simulink model "OSWEC"  (R2020a)
settings: Solver=ode4  StartTime=0  StopTime=200  FixedStep=0.01  MaxStep=0.01  RelTol=1e-3  EnableMultiTasking=on
values from neighbouring files (symbols this model uses):
  Bv = viscLDamp + ptoDamp + viscQDamp    [ptoSimInputFile.m]    (also in userDefinedFunctions.m)
  controller = struct()    [ptoSimInputFile.m]
  ptosim = ptoSimClass('Non-Compressible Fluid Hydraulic')    [ptoSimInputFile.m]
  R = body(1).hydroData.hydro_coeffs.radiation_damping.all(5,5,w_ind).*simu.rho*2*pi/waves.T    [ptoSimInputFile.m]    (also in userDefinedFunctions.m)
  simu = simulationClass()    [wecSimInputFile.m]
  waves = waveClass('irregular')    [wecSimInputFile.m]
undefined symbols (not defined in the file or in its folder): body, constraint, pto, X, Y, Z
libraries: nesl_utility x22, sm_lib x16, WECSim_Lib x10, PTOSim_Lib x3, vrlib x1, simulink x1
(part 3 of 4)

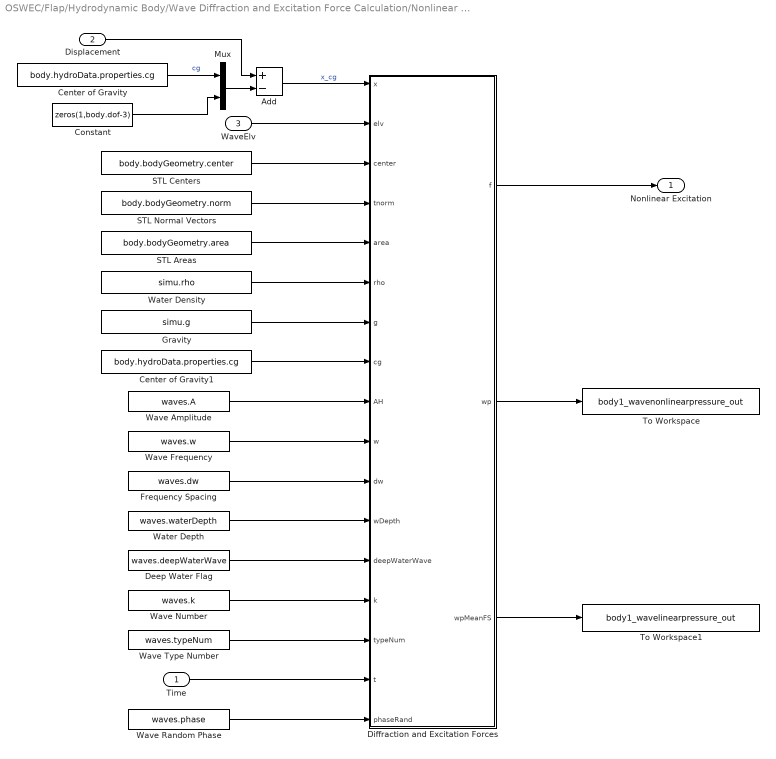
== system OSWEC/Flap/Hydrodynamic Body/Wave Diffraction and Excitation Force Calculation/Nonlinear FK Force Variant Subsystem/With Nonlinear FroudeKrylov Force ==
  Time : Inport
  Displacement : Inport  Port=2
  WaveElv : Inport  Port=3
  Add : Sum  Inputs=+-
  Center of Gravity : Constant  Value=body.hydroData.properties.cg
  Center of Gravity1 : Constant  Value=body.hydroData.properties.cg
  Constant : Constant  Value=zeros(1,body.dof-3)
  Deep Water Flag : Constant  Value=waves.deepWaterWave
  Diffraction and Excitation Forces : MATLAB Function  TreatAsAtomicUnit=on
  Frequency Spacing : Constant  Value=waves.dw
  Gravity : Constant  Value=simu.g
  Mux : Mux  Inputs=2
  STL Areas : Constant  Value=body.bodyGeometry.area
  STL Centers : Constant  Value=body.bodyGeometry.center
  STL Normal Vectors : Constant  Value=body.bodyGeometry.norm
  To Workspace : ToWorkspace  VariableName=body1_wavenonlinearpressure_out  SaveFormat=Structure With Time  SampleTime=-1
      settings: Decimation=round(simu.dtOut/simu.dt,0)
  To Workspace1 : ToWorkspace  VariableName=body1_wavelinearpressure_out  SaveFormat=Structure With Time  SampleTime=-1
      settings: Decimation=round(simu.dtOut/simu.dt,0)
  Water Density : Constant  Value=simu.rho
  Water Depth : Constant  Value=waves.waterDepth
  Wave Amplitude : Constant  Value=waves.A
  Wave Frequency : Constant  Value=waves.w
  Wave Number : Constant  Value=waves.k
  Wave Random Phase : Constant  Value=waves.phase
  Wave Type Number : Constant  Value=waves.typeNum
  Nonlinear Excitation : Outport
  wires:
  STL Areas/1 -> Diffraction and Excitation Forces/5(area)
  Diffraction and Excitation Forces/2(wp) -> To Workspace/1
  Diffraction and Excitation Forces/3(wpMeanFS) -> To Workspace1/1
  Displacement/1 -> Add/1
  Constant/1 -> Mux/2
  Center of Gravity/1 -> Mux/1  "cg"
  Mux/1 -> Add/2
  Add/1 -> Diffraction and Excitation Forces/1(x)  "x_cg"
  Deep Water Flag/1 -> Diffraction and Excitation Forces/13(deepWaterWave)
  Wave Random Phase/1 -> Diffraction and Excitation Forces/17(phaseRand)
  Water Depth/1 -> Diffraction and Excitation Forces/12(wDepth)
  Wave Number/1 -> Diffraction and Excitation Forces/14(k)
  Wave Type Number/1 -> Diffraction and Excitation Forces/15(typeNum)
  Frequency Spacing/1 -> Diffraction and Excitation Forces/11(dw)
  Wave Frequency/1 -> Diffraction and Excitation Forces/10(w)
  Wave Amplitude/1 -> Diffraction and Excitation Forces/9(AH)
  Time/1 -> Diffraction and Excitation Forces/16(t)
  WaveElv/1 -> Diffraction and Excitation Forces/2(elv)
  STL Centers/1 -> Diffraction and Excitation Forces/3(center)
  STL Normal Vectors/1 -> Diffraction and Excitation Forces/4(tnorm)
  Water Density/1 -> Diffraction and Excitation Forces/6(rho)
  Gravity/1 -> Diffraction and Excitation Forces/7(g)
  Diffraction and Excitation Forces/1(f) -> Nonlinear Excitation/1
  Center of Gravity1/1 -> Diffraction and Excitation Forces/8(cg)

== system OSWEC/Flap/Hydrodynamic Body/Wave Radiation Forces Calculation/SS CI and Constant-Damping-CoeVariant Subsystem/Constant Coefficients ==
  note: F = damping * velocity
  velocity : Inport
  Product : Product  Multiplication=Matrix(*)
  Radiation Damping Matrix : Constant  Value=body.hydroForce.fDamping
  Out1 : Outport
  wires:
  velocity/1 -> Product/2
  Product/1 -> Out1/1  "F_Single Frequency"
  Radiation Damping Matrix/1 -> Product/1

== system OSWEC/Flap/Hydrodynamic Body/Wave Radiation Forces Calculation/SS CI and Constant-Damping-CoeVariant Subsystem/Convolution Integral Calculation ==
  note: Calculate the convolution integral using the radiation IRF (body.hydroForce.irkb) and the velocity.
  velocity : Inport
  CTTime : Constant  Value=simu.CTTime
  IRBK : Constant  Value=body.hydroForce.irkb
  MATLAB Function1 : MATLAB Function  TreatAsAtomicUnit=on  SystemSampleTime=simu.CTTime(2)-simu.CTTime(1)
  Rate Transition : RateTransition
  Reshape : Reshape
  Out1 : Outport
  wires:
  velocity/1 -> MATLAB Function1/1(velocity)
  CTTime/1 -> MATLAB Function1/3(CTTime)
  IRBK/1 -> MATLAB Function1/2(IRKB)
  MATLAB Function1/1(F_FM) -> Rate Transition/1
  Rate Transition/1 -> Reshape/1
  Reshape/1 -> Out1/1

== system OSWEC/Flap/Hydrodynamic Body/Wave Radiation Forces Calculation/SS CI and Constant-Damping-CoeVariant Subsystem/State-Space Calculation  ==
  note: Calculate the radiation damping based on the state space formulation. Coefficients are defined in body.hydroForce.ssRadf
  velocity : Inport
  State-Space : StateSpace  A=body.hydroForce.ssRadf.A  B=body.hydroForce.ssRadf.B  C=body.hydroForce.ssRadf.C  D=body.hydroForce.ssRadf.D  InitialCondition=0
  Out1 : Outport
  wires:
  State-Space/1 -> Out1/1
  velocity/1 -> State-Space/1  "x"

== system OSWEC/controller(1)/Rotary to Linear Adjustable Rod1/Angle Calculation for PTO/Subsystem1/Distance btw flap joint & rod joint along x-axis ==
  Add3 : Sum  Inputs=+-
  Add4 : Sum  Inputs=+-
  Constant1 : Constant  Value=ptosim.crank
  Constant2 : Constant  Value=ptosim.rodInit
  Constant3 : Constant  Value=ptosim.offset
  Math Function2 : Math  Operator=square  SignedPower=on  SaturateOnIntegerOverflow=on
  Math Function3 : Math  Operator=square  SignedPower=on  SaturateOnIntegerOverflow=on
  Sqrt1 : Sqrt  SaturateOnIntegerOverflow=on
  d : Outport
  wires:
  Add3/1 -> Sqrt1/1
  Constant2/1 -> Math Function2/1
  Constant1/1 -> Add4/1
  Constant3/1 -> Add4/2
  Add4/1 -> Math Function3/1
  Math Function3/1 -> Add3/2
  Math Function2/1 -> Add3/1
  Sqrt1/1 -> d/1

== system OSWEC/controller(1)/Rotary to Linear Adjustable Rod1/Angle Calculation for PTO/Subsystem2/Distance btw flap joint & rod joint along x-axis ==
  Add3 : Sum  Inputs=+-
  Add4 : Sum  Inputs=+-
  Constant1 : Constant  Value=ptosim.crank
  Constant2 : Constant  Value=ptosim.rodInit
  Constant3 : Constant  Value=ptosim.offset
  Math Function2 : Math  Operator=square  SignedPower=on  SaturateOnIntegerOverflow=on
  Math Function3 : Math  Operator=square  SignedPower=on  SaturateOnIntegerOverflow=on
  Sqrt1 : Sqrt  SaturateOnIntegerOverflow=on
  d : Outport
  wires:
  Add3/1 -> Sqrt1/1
  Constant2/1 -> Math Function2/1
  Constant1/1 -> Add4/1
  Constant3/1 -> Add4/2
  Add4/1 -> Math Function3/1
  Math Function3/1 -> Add3/2
  Math Function2/1 -> Add3/1
  Sqrt1/1 -> d/1

== system OSWEC/controller(1)/Rotary to Linear Adjustable Rod1/Angular to Linear Velocity/Subsystem/Distance btw flap joint & rod joint along x-axis ==
  Add3 : Sum  Inputs=+-
  Add4 : Sum  Inputs=+-
  Constant4 : Constant  Value=ptosim.rodInit
  Constant5 : Constant  Value=ptosim.crank
  Constant6 : Constant  Value=ptosim.offset
  Math Function2 : Math  Operator=square  SignedPower=on  SaturateOnIntegerOverflow=on
  Math Function3 : Math  Operator=square  SignedPower=on  SaturateOnIntegerOverflow=on
  Sqrt1 : Sqrt  SaturateOnIntegerOverflow=on
  d : Outport
  wires:
  Sqrt1/1 -> d/1
  Math Function2/1 -> Add3/1
  Math Function3/1 -> Add3/2
  Add4/1 -> Math Function3/1
  Constant6/1 -> Add4/2
  Constant5/1 -> Add4/1
  Constant4/1 -> Math Function2/1
  Add3/1 -> Sqrt1/1

== system OSWEC/Flap/Hydrodynamic Body/Hydrostatic Restoring Force Calculation/Linear and Nonlinear Restoring Force Variant Subsystem/Linear Hydrostatic Restoring Force /Net Buoyancy Force ==
  note: The total buoyancy force is due to the vertical buoyancy force (gravity - buoyancy) and a rotational buoyancy force if the center of gravity is not aligned with the center of buoyancy.
      |
      | F_NetBuoyancy = F_gravity - F_buoyancy + F_rotational_buoyancy
      |
      | F_rotational_buoyancy = (cb-cg) x F_buoyancy
      | F_buoyancy = rho*g*V_0
      | F_gravity = m*g
  Body Mass : Inport
  Add1 : Sum  Inputs=+-
  Add2 : Sum
  Add3 : Sum  Inputs=+-
  Assignment (Add Net Bouyancy Force to Z-Direction) : Assignment  IndexOptions=Index vector (dialog)  Indices=3  OutputSizes=1
  Assignment (Add Net Bouyancy Force to Z-Direction)1 : Assignment  IndexOptions=Index vector (dialog)  Indices=3  OutputSizes=1
  Assignment (Add Net Bouyancy Force to Z-Direction)2 : Assignment  IndexOptions=Index vector (dialog)  Indices=4:6  OutputSizes=1
  Center of Buoyancy : Constant  Value=body.cb
  Center of Gravity : Constant  Value=body.cg
  Constant1 : Constant  Value=zeros(1,body.dof)
  Constant2 : Constant  Value=[0 0 0]
  Cross Product : vrlib/Utilities/Cross Product
  Gravity : Constant  Value=simu.g
  Product : Product
  Product1 : Product  Inputs=3
  Volume : Constant  Value=body.dispVol
  Water Density : Constant  Value=simu.rho
  F_NetBuoyancy : Outport
  wires:
  Add1/1 -> Assignment (Add Net Bouyancy Force to Z-Direction)/2
  Body Mass/1 -> Product/2  "m"
  Cross Product/1 -> Assignment (Add Net Bouyancy Force to Z-Direction)2/2
  Add2/1 -> F_NetBuoyancy/1  "Net buoyancy force"
  Add3/1 -> Cross Product/2
  Constant2/1 -> Assignment (Add Net Bouyancy Force to Z-Direction)1/1
  Center of Gravity/1 -> Add3/2  "cg"
  Constant1/1 -> Assignment (Add Net Bouyancy Force to Z-Direction)/1, Assignment (Add Net Bouyancy Force to Z-Direction)2/1
  Center of Buoyancy/1 -> Add3/1  "x"
  Assignment (Add Net Bouyancy Force to Z-Direction)1/1 -> Cross Product/1
  Volume/1 -> Product1/3  "Vol"
  Assignment (Add Net Bouyancy Force to Z-Direction)/1 -> Add2/1  "Vertical Buoyancy Force"
  Water Density/1 -> Product1/1  "rho"
  Gravity/1 -> Product/1, Product1/2  "g"
  Product1/1 -> Assignment (Add Net Bouyancy Force to Z-Direction)1/2, Add1/2  "F_Buoyancy"
  Product/1 -> Add1/1  "F_Gravity"
  Assignment (Add Net Bouyancy Force to Z-Direction)2/1 -> Add2/2  "Rotational buoyancy force"

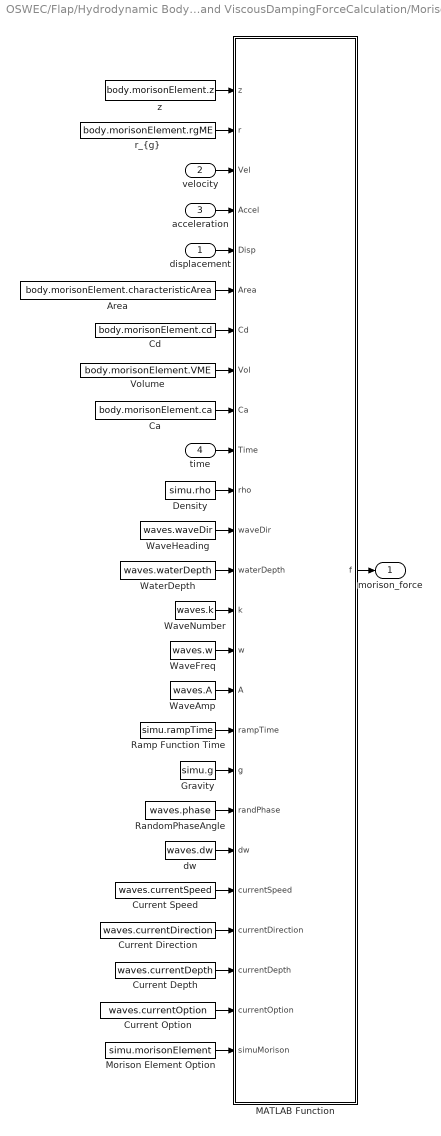
== system OSWEC/Flap/Hydrodynamic Body/Morison Element and ViscousDampingForceCalculation/Morison Element Variant Subsystem/Morison Element On/Irregular Wave Morison Force ==
  displacement : Inport
  velocity : Inport  Port=2
  acceleration : Inport  Port=3
  time : Inport  Port=4
  Area : Constant  Value=body.morisonElement.characteristicArea  VectorParams1D=off
  Ca : Constant  Value=body.morisonElement.ca  VectorParams1D=off
  Cd : Constant  Value=body.morisonElement.cd  VectorParams1D=off
  Current Depth : Constant  Value=waves.currentDepth
  Current Direction : Constant  Value=waves.currentDirection
  Current Option : Constant  Value=waves.currentOption
  Current Speed : Constant  Value=waves.currentSpeed
  Density : Constant  Value=simu.rho
  Gravity : Constant  Value=simu.g
  MATLAB Function : MATLAB Function  TreatAsAtomicUnit=on
  Morison Element Option : Constant  Value=simu.morisonElement
  Ramp Function Time : Constant  Value=simu.rampTime
  RandomPhaseAngle : Constant  Value=waves.phase  VectorParams1D=off
  Volume : Constant  Value=body.morisonElement.VME  VectorParams1D=off
  WaterDepth : Constant  Value=waves.waterDepth
  WaveAmp : Constant  Value=waves.A
  WaveFreq : Constant  Value=waves.w
  WaveHeading : Constant  Value=waves.waveDir
  WaveNumber : Constant  Value=waves.k
  dw : Constant  Value=waves.dw  VectorParams1D=off
  "r_{g}" : Constant  Value=body.morisonElement.rgME  VectorParams1D=off
  z : Constant  Value=body.morisonElement.z  VectorParams1D=off
  morison_force : Outport
  wires:
  Morison Element Option/1 -> MATLAB Function/25(simuMorison)
  Current Option/1 -> MATLAB Function/24(currentOption)
  Current Depth/1 -> MATLAB Function/23(currentDepth)
  Current Direction/1 -> MATLAB Function/22(currentDirection)
  Current Speed/1 -> MATLAB Function/21(currentSpeed)
  dw/1 -> MATLAB Function/20(dw)
  RandomPhaseAngle/1 -> MATLAB Function/19(randPhase)
  Gravity/1 -> MATLAB Function/18(g)
  Ramp Function Time/1 -> MATLAB Function/17(rampTime)
  WaveAmp/1 -> MATLAB Function/16(A)
  WaveFreq/1 -> MATLAB Function/15(w)
  WaveNumber/1 -> MATLAB Function/14(k)
  WaterDepth/1 -> MATLAB Function/13(waterDepth)
  WaveHeading/1 -> MATLAB Function/12(waveDir)
  Density/1 -> MATLAB Function/11(rho)
  time/1 -> MATLAB Function/10(Time)
  Ca/1 -> MATLAB Function/9(Ca)
  Volume/1 -> MATLAB Function/8(Vol)
  Cd/1 -> MATLAB Function/7(Cd)
  Area/1 -> MATLAB Function/6(Area)
  displacement/1 -> MATLAB Function/5(Disp)
  acceleration/1 -> MATLAB Function/4(Accel)
  velocity/1 -> MATLAB Function/3(Vel)
  "r_{g}"/1 -> MATLAB Function/2(r)
  z/1 -> MATLAB Function/1(z)
  MATLAB Function/1(f) -> morison_force/1

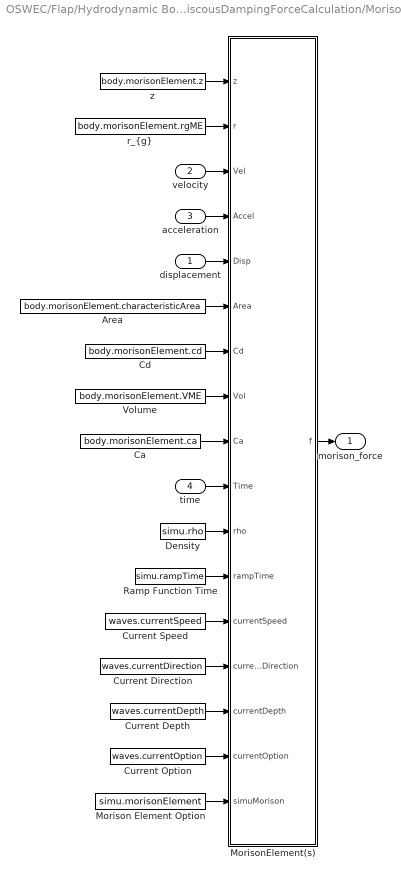
== system OSWEC/Flap/Hydrodynamic Body/Morison Element and ViscousDampingForceCalculation/Morison Element Variant Subsystem/Morison Element On/No Wave Morison Force ==
  displacement : Inport
  velocity : Inport  Port=2
  acceleration : Inport  Port=3
  time : Inport  Port=4
  Area : Constant  Value=body.morisonElement.characteristicArea  VectorParams1D=off
  Ca : Constant  Value=body.morisonElement.ca  VectorParams1D=off
  Cd : Constant  Value=body.morisonElement.cd  VectorParams1D=off
  Current Depth : Constant  Value=waves.currentDepth
  Current Direction : Constant  Value=waves.currentDirection
  Current Option : Constant  Value=waves.currentOption
  Current Speed : Constant  Value=waves.currentSpeed
  Density : Constant  Value=simu.rho
  Morison Element Option : Constant  Value=simu.morisonElement
  MorisonElement(s) : MATLAB Function  TreatAsAtomicUnit=on
  Ramp Function Time : Constant  Value=simu.rampTime
  Volume : Constant  Value=body.morisonElement.VME  VectorParams1D=off
  "r_{g}" : Constant  Value=body.morisonElement.rgME  VectorParams1D=off
  z : Constant  Value=body.morisonElement.z  VectorParams1D=off
  morison_force : Outport
  wires:
  Morison Element Option/1 -> MorisonElement(s)/17(simuMorison)
  Current Option/1 -> MorisonElement(s)/16(currentOption)
  Current Depth/1 -> MorisonElement(s)/15(currentDepth)
  Current Direction/1 -> MorisonElement(s)/14(currentDirection)
  Current Speed/1 -> MorisonElement(s)/13(currentSpeed)
  Ramp Function Time/1 -> MorisonElement(s)/12(rampTime)
  Density/1 -> MorisonElement(s)/11(rho)
  time/1 -> MorisonElement(s)/10(Time)
  Ca/1 -> MorisonElement(s)/9(Ca)
  Volume/1 -> MorisonElement(s)/8(Vol)
  Cd/1 -> MorisonElement(s)/7(Cd)
  Area/1 -> MorisonElement(s)/6(Area)
  displacement/1 -> MorisonElement(s)/5(Disp)
  acceleration/1 -> MorisonElement(s)/4(Accel)
  velocity/1 -> MorisonElement(s)/3(Vel)
  "r_{g}"/1 -> MorisonElement(s)/2(r)
  z/1 -> MorisonElement(s)/1(z)
  MorisonElement(s)/1(f) -> morison_force/1

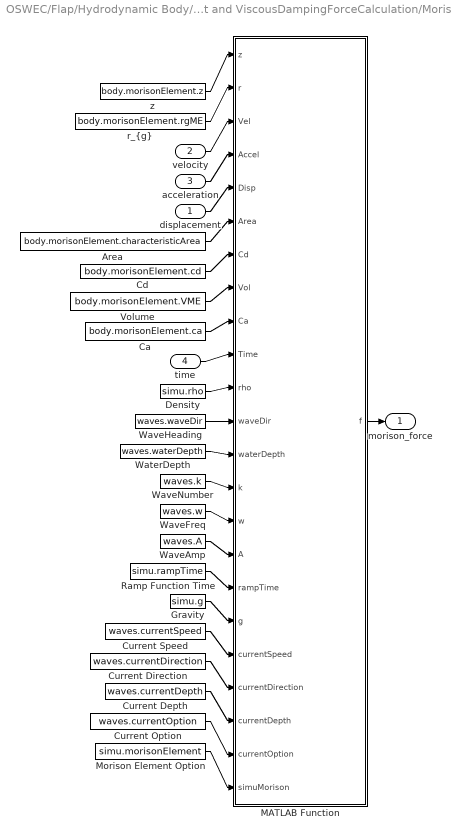
== system OSWEC/Flap/Hydrodynamic Body/Morison Element and ViscousDampingForceCalculation/Morison Element Variant Subsystem/Morison Element On/Regular Wave Morison Force ==
  displacement : Inport
  velocity : Inport  Port=2
  acceleration : Inport  Port=3
  time : Inport  Port=4
  Area : Constant  Value=body.morisonElement.characteristicArea  VectorParams1D=off
  Ca : Constant  Value=body.morisonElement.ca  VectorParams1D=off
  Cd : Constant  Value=body.morisonElement.cd  VectorParams1D=off
  Current Depth : Constant  Value=waves.currentDepth
  Current Direction : Constant  Value=waves.currentDirection
  Current Option : Constant  Value=waves.currentOption
  Current Speed : Constant  Value=waves.currentSpeed
  Density : Constant  Value=simu.rho
  Gravity : Constant  Value=simu.g
  MATLAB Function : MATLAB Function  TreatAsAtomicUnit=on
  Morison Element Option : Constant  Value=simu.morisonElement
  Ramp Function Time : Constant  Value=simu.rampTime
  Volume : Constant  Value=body.morisonElement.VME  VectorParams1D=off
  WaterDepth : Constant  Value=waves.waterDepth
  WaveAmp : Constant  Value=waves.A
  WaveFreq : Constant  Value=waves.w
  WaveHeading : Constant  Value=waves.waveDir
  WaveNumber : Constant  Value=waves.k
  "r_{g}" : Constant  Value=body.morisonElement.rgME  VectorParams1D=off
  z : Constant  Value=body.morisonElement.z  VectorParams1D=off
  morison_force : Outport
  wires:
  Current Speed/1 -> MATLAB Function/19(currentSpeed)
  WaveAmp/1 -> MATLAB Function/16(A)
  Gravity/1 -> MATLAB Function/18(g)
  WaveNumber/1 -> MATLAB Function/14(k)
  Ca/1 -> MATLAB Function/9(Ca)
  Current Direction/1 -> MATLAB Function/20(currentDirection)
  Area/1 -> MATLAB Function/6(Area)
  WaterDepth/1 -> MATLAB Function/13(waterDepth)
  acceleration/1 -> MATLAB Function/4(Accel)
  Density/1 -> MATLAB Function/11(rho)
  WaveHeading/1 -> MATLAB Function/12(waveDir)
  WaveFreq/1 -> MATLAB Function/15(w)
  Cd/1 -> MATLAB Function/7(Cd)
  displacement/1 -> MATLAB Function/5(Disp)
  Current Option/1 -> MATLAB Function/22(currentOption)
  Current Depth/1 -> MATLAB Function/21(currentDepth)
  time/1 -> MATLAB Function/10(Time)
  "r_{g}"/1 -> MATLAB Function/2(r)
  Ramp Function Time/1 -> MATLAB Function/17(rampTime)
  velocity/1 -> MATLAB Function/3(Vel)
  Volume/1 -> MATLAB Function/8(Vol)
  Morison Element Option/1 -> MATLAB Function/23(simuMorison)
  z/1 -> MATLAB Function/1(z)
  MATLAB Function/1(f) -> morison_force/1

== matlab function OSWEC/Flap/Hydrodynamic Body/Morison Element and ViscousDampingForceCalculation/Morison Element Variant Subsystem/Morison Element On/Irregular Wave Morison Force/MATLAB Function ==
  data: z input; f output; r input; Vel input; Accel input; Disp input; Area input; Cd input; Vol input; Ca input; Time input; rho input; waveDir input; waterDepth input; k input; w input; A input; rampTime input; g input; randPhase input; dw input; currentSpeed input; currentDirection input; currentDepth input; currentOption input; simuMorison input
function f = fcn(z,r,Vel,Accel,Disp,Area,Cd,Vol,Ca,Time,rho,waveDir,waterDepth,k,w,A,rampTime,g,randPhase,dw,currentSpeed,currentDirection,currentDepth,currentOption,simuMorison)
% This function calculates the Morison element force for the irregular wave
% case.
[rr,~]  = size(r); [ff]    = length(w);
FMt     = zeros(rr,6);
uVt     = zeros(ff,1); vVt = uVt; wVt = vVt; uAt = wVt; vAt = uAt; wAt = vAt;
for ii = 1:rr
    % Calculate Rotation Matrix
    RotMax = [cos(Disp(5))*cos(Disp(6)) , cos(Disp(4))*sin(Disp(6)) + sin(Disp(4))*sin(Disp(5))*cos(Disp(6)) , sin(Disp(4))*sin(Disp(6)) - cos(Disp(4))*sin(Disp(5))*sin(Disp(6));...
              -cos(Disp(5))*sin(Disp(6)), cos(Disp(4))*cos(Disp(6)) -  sin(Disp(4))*sin(Disp(5))*sin(Disp(6)), sin(Disp(4))*cos(Disp(6)) + cos(Disp(4))*sin(Disp(5))*sin(Disp(6));...
              sin(Disp(5))              , -sin(Disp(4))*cos(Disp(5))                                         , cos(Disp(4))*cos(Disp(5))                                        ];
    % Rotate Cartesian
    rRot    = mtimes(RotMax,r(ii,:).')';
    Dispt   = [Disp(1),Disp(2),Disp(3)];
    ShiftCg = Dispt + rRot;
    zRot    = mtimes(RotMax,z(ii,:)')';
    % Update translational and rotational velocity
    % w refers to \omega = rotational velocity
    Velt    = [Vel(4),Vel(5),Vel(6)];
    wxr     = cross(Velt,r(ii,:));
    %
    switch currentOption
        case 0
            currentSpeedDepth = currentSpeed;
        case 1
            if ShiftCg(3) > -currentDepth
                currentSpeedDepth = currentSpeed*(1 + ShiftCg(3)/currentDepth)^(1/7);
            else
                currentSpeedDepth = 0;
            end
        case 2
            if ShiftCg(3) > -currentDepth
                currentSpeedDepth = currentSpeed*(1 + ShiftCg(3)/currentDepth);
            else
                currentSpeedDepth = 0;
            end
        otherwise
            currentSpeedDepth = 0;
    end
    % Ramp Time
    if Time <= rampTime
        curramp        = currentSpeedDepth*(1 + cos(pi + pi/rampTime*Time))/2;
    else
        curramp        = currentSpeedDepth;
    end
    %Vel should be a column vector
    Vel2    = [Vel(1),Vel(2),Vel(3)] + wxr + [curramp*cosd(currentDirection),curramp*sind(currentDirection),0];
    % Update translational and rotational acceleration
    % dotw refers to \dot{\omega} = rotational acceleration
    Accelt  = [Accel(4),Accel(5),Accel(6)];
    dotwxr  = cross(Accelt,r(ii,:));
    wxwxr   = cross(Velt,wxr);
    % Update Translational Acceleration
    Accel2  = [Accel(1),Accel(2),Accel(3)] + dotwxr + wxwxr;
    %% Calculate Orbital Velocity
    for jj = 1:ff
        waveDirRad      = waveDir*pi/180;
        phaseArg        = w(jj,1)*Time - k(jj,1)*(ShiftCg(1)*cos(waveDirRad) + ShiftCg(2)*sin(waveDirRad)) + randPhase(jj,1);
        % Vertical Variation
        kh              = k(jj,1)*waterDepth;
        kz              = k(jj,1)*ShiftCg(3);
        if kh > pi 
            % Deep Water Wave Assumption
            coeffHorz  = exp(kz);
            coeffVert  = coeffHorz;
        else
            % Shallow & Intermediate depth
            coeffHorz  = cosh(kz + kh)/cosh(kh);
            coeffVert  = sinh(kz + kh)/cosh(kh);
        end
        % Ramp Time
        if Time <= rampTime
            ramp        = (sqrt(A(jj,1)*dw(jj,1))/2)*(1 + cos(pi + pi/rampTime*Time));
        else
            ramp        = sqrt(A(jj,1)*dw(jj,1));
        end
        % Orbital Velocity for each individual wave component
        uVt(jj,1)       =  ramp*coeffHorz*cos(phaseArg)*g*k(jj,1)*(1/w(jj,1))*cos(waveDirRad);
        vVt(jj,1)       =  ramp*coeffHorz*cos(phaseArg)*g*k(jj,1)*(1/w(jj,1))*sin(waveDirRad);
        wVt(jj,1)       = -ramp*coeffVert*sin(phaseArg)*g*k(jj,1)*(1/w(jj,1));
        % Orbital Acceleration for each individual wave component
        uAt(jj,1)       = -ramp*coeffHorz*sin(phaseArg)*g*k(jj,1)*cos(waveDirRad);
        vAt(jj,1)       = -ramp*coeffHorz*sin(phaseArg)*g*k(jj,1)*sin(waveDirRad);
        wAt(jj,1)       = -ramp*coeffVert*cos(phaseArg)*g*k(jj,1);
    end
    % Sum the wave components to obtain the x, y, z orbital velocities
    uV = sum(uVt); uA   = sum(uAt); vV = sum(vVt); vA = sum(vAt); wV = sum(wVt); wA = sum(wAt);
    fluidV              = [uV, vV, wV];
    fluidA              = [uA, vA, wA];
    if simuMorison == 2
        %% Decompose Fluid Velocity
        % Tangential Velocity
        vT              = ((dot(zRot,fluidV))/(norm(zRot)^2))*zRot;        
        % Normal Velocity
        vN              = fluidV-vT;
        %% Decompose Fluid Acceleration
        AT              = ((dot(zRot,fluidA))/(norm(zRot)^2))*zRot;        
        % Normal Acceleration
        AN              = fluidA-AT;
        %% Decompose Body Velocity
        % Tangential Velocity
        Vel2T           = ((dot(zRot,Vel2))/(norm(zRot)^2))*zRot;       
        % Normal Velocity
        Vel2N           = Vel2-Vel2T;
        %% Decompose Body Acceleration
        Accel2T         = ((dot(zRot,Accel2))/(norm(zRot)^2))*zRot;   
        % Normal Acceleration
        Accel2N         = Accel2-Accel2T;
        %% Morison Equation
        % Forces from velocity drag
        FdN             = (1/2)*rho*Cd(ii,1)*Area(ii,1)*(vN-Vel2N)*norm(vN-Vel2N);                               
        FdT             = (1/2)*rho*Cd(ii,2)*Area(ii,2)*(vT-Vel2T)*norm(vT-Vel2T);                                          
        Fd              = FdT + FdN;
        % Forces from body acceleration inertia on the Morison Element
        FiN             = rho*Vol(ii,:)*Ca(ii,1)*(AN - Accel2N);            % AdiffN;
        FiT             = rho*Vol(ii,:)*Ca(ii,2)*(AT - Accel2T);            % AdiffT;
        Fbi             = FiN + FiT;
        % Forces from fluid acceleration inertia on the Morison Element
        Ffi             = rho*Vol(ii,:)*(fluidA);
        % Summation of inertial forces on the Morison Element
        Fi              = Ffi + Fbi;
        % Total Force from the Morison Element
        F               = Fi + Fd;
    else
        %% Added inertia and drag forces
        areaRot         = abs(mtimes(Area(ii,:),RotMax));
        CdRot           = mtimes(abs(Cd(ii,:)),RotMax);
        CaRot           = abs(mtimes(Ca(ii,:),RotMax));
        % Forces from velocity drag
        uVdiff          = uV - Vel2(1); FxuV = (1/2)*abs(uVdiff)*uVdiff*rho*CdRot(1)*areaRot(1);
        vVdiff          = vV - Vel2(2); FxvV = (1/2)*abs(vVdiff)*vVdiff*rho*CdRot(2)*areaRot(2);
        wVdiff          = wV - Vel2(3); FxwV = (1/2)*abs(wVdiff)*wVdiff*rho*CdRot(3)*areaRot(3);
        % Forces from body acceleration inertia
        uAdiff          = uA - Accel2(1); FxuA = uAdiff*rho*Vol(ii,:)*CaRot(1);
        vAdiff          = vA - Accel2(2); FxvA = vAdiff*rho*Vol(ii,:)*CaRot(2);
        wAdiff          = wA - Accel2(3); FxwA = wAdiff*rho*Vol(ii,:)*CaRot(3);
        % Forces from fluid acceleration inertia
        FxuAf           = uA*Vol(ii,:)*rho;
        FxvAf           = vA*Vol(ii,:)*rho;
        FxwAf           = wA*Vol(ii,:)*rho;
        % Total Force from the Morison Element
        F               = [FxuV + FxuA + FxuAf,...
                           FxvV + FxvA + FxvAf,...
                           FxwV + FxwA + FxwAf];
    end
    % Determine if the Morison Element point of application goes above the
    % mean water line and does not consider the local surface elevation.
    if ShiftCg(3) > 0
        F           = [0, 0, 0];
        M           = [0, 0, 0];
        FMt(ii,:)   = [F,M];
    else
        % Calculate the moment about the center of gravity for each Morison Element
        M           = cross(rRot,F);
        FMt(ii,:)   = [F,M];
    end
end
f      = 0.* Vel;
f(1:6) = [sum(FMt(:,1));sum(FMt(:,2));sum(FMt(:,3));sum(FMt(:,4));sum(FMt(:,5));sum(FMt(:,6))];

== matlab function OSWEC/Flap/Hydrodynamic Body/Nonlinear Wave Elevation/Linear or Instantaneous Free Surface/Instantaneous Water Free Surface  /Instantaneous FS ==
  data: x input; center input; f output; cg input; AH input; w input; dw input; k input; typeNum input; t input; rampT input; phaseRand input; waveDir input
function f  = waveElevation(x,center,cg,AH,w,dw,k,typeNum,t,rampT,phaseRand,waveDir)
% Function to calculate the wave elevation at the ceontroids of triangulated surface
% NOTE: This function assumes that the STL file is imported with its CG at 0,0,0
f = calc_elev(x,center,cg,AH,w,dw,k,typeNum,t,rampT,phaseRand, waveDir);
end

function f = calc_elev(x,center,cg,AH,w,dw,k,typeNum,t,rampT,phaseRand,waveDir)
% Function to rotate and translate body and call wave elevation function at new locations

% Compute new tri center coords after cog rotation and translation
center = rotateXYZ(center,[1 0 0],x(4));
center = rotateXYZ(center,[0 1 0],x(5));
center = rotateXYZ(center,[0 0 1],x(6));
center = offsetXYZ(center,x);
center = offsetXYZ(center,cg);
% Calculate the free surface
f=waveElev(center,AH,w,dw,t,k,rampT,phaseRand,typeNum,waveDir);
end

function f=waveElev(center,AH,w,dw,t,k,rampT,phaseRand,typeNum,waveDir)
% Function to calculate the wave elevation at an array of points
f = zeros(length(center(:,3)),1);
cx = center(:,1);
cy = center(:,2);
X = cx*cos(waveDir*pi/180) + cy*sin(waveDir*pi/180);
if typeNum <10
elseif typeNum <20
    f = AH(1).*cos(k(1).*X-w(1)*t);
elseif typeNum <30
    tmp=sqrt(AH.*dw);
    tmp1 = ones(1,length(center(:,1)));
    tmp2 = (w.*t+phaseRand)*tmp1;
    tmp3 = cos(k*X'- tmp2);
    f(:,1) = tmp3'*tmp;
end
if t<=rampT
    rampF = (1+cos(pi+pi*t/rampT))/2;
    f = f.*rampF;
end
end

== matlab function OSWEC/Flap/Hydrodynamic Body/Structure/Motion Sensor/quaternion2EulXYZ ==
  data: Q input; E output
function E = fcn(Q)
% Call quaternion matlab function. 
% Saved as separate text file for Github tracking purposes.
% Can't use MATLAB interpreted function because they don't allow for code 
% generation (used in rapid accelerator mode)
E = quaternion2EulXYZ(Q);
end

== matlab function OSWEC/Flap/Hydrodynamic Body/Wave Diffraction and Excitation Force Calculation/Linear Wave Excitation Force Variant Subsystem/Irregular Wave Excitation Force/MATLAB Function ==
  data: A input; Fext output; w input; fExtRE input; fExtIM input; phaseRand input; dw input; time input; WaveDir input; WaveSpread input; fExtMD input
function Fext = fcn(A,w,fExtRE,fExtIM,phaseRand,dw,time,WaveDir,WaveSpread,fExtMD)
%#codegen

% pversistent A1 B1 B11 C1 D1 D11 E1 E11

A1=bsxfun(@plus,w*time,pi/2);
%Fext = zeros(1,6);
Fext = zeros(1,size(fExtRE,3));
for ii=1:length(WaveDir)
    B1= sin(bsxfun(@plus,A1,phaseRand(:,ii)));
    B11 = sin(bsxfun(@plus,w*time,phaseRand(:,ii)));
    C0 = bsxfun(@times,A*WaveSpread(ii),dw);
    C1 = sqrt(bsxfun(@times,A*WaveSpread(ii),dw));
    D0 =bsxfun(@times,squeeze(fExtMD(ii,:,:)),C0);
    D1 =bsxfun(@times,squeeze(fExtRE(ii,:,:)),C1);
    D11 = bsxfun(@times,squeeze(fExtIM(ii,:,:)),C1);
    E1 = D0+ bsxfun(@times,B1,D1);
    E11 = bsxfun(@times,B11,D11);
    Fext = Fext + sum(bsxfun(@minus,E1,E11));
end

== matlab function OSWEC/Flap/Hydrodynamic Body/Wave Diffraction and Excitation Force Calculation/Nonlinear FK Force Variant Subsystem/With Nonlinear FroudeKrylov Force/Diffraction and Excitation Forces ==
  data: x input; elv input; center input; f output; tnorm input; area input; rho input; g input; cg input; AH input; w input; dw input; wDepth input; deepWaterWave input; k input; typeNum input; t input; phaseRand input; wp output; wpMeanFS output
function [f, wp, wpMeanFS]  = nonFKForce(x,elv,center,tnorm,area,rho,g,cg,AH,w,dw,wDepth,deepWaterWave,k,typeNum,t,phaseRand)
% Function to calculate the wave excitation force and moment on a
% triangulated surface. The nonlinear excitation forces are calculated by
% intergrating the pressure over the triangulated surface and subtracting
% the linear excitation force (this is added back in later):
%    F_exc_nonlinear = F_exc_total - F_exc_linear
% NOTE: This function assumes that the STL file is imported with its CG at 0,0,0

% Logic to calculate nonFKForce at reduced sample time
[f, wp, wpMeanFS] = calc_force(x,elv,center,tnorm,area,rho,g,cg,AH,w,dw,wDepth,deepWaterWave,k,typeNum,t,phaseRand);
end

function [f, wp, wpMeanFS]  = calc_force(x,elv,center,tnorm,area,rho,g,cg,AH,w,dw,wDepth,deepWaterWave,k,typeNum,t,phaseRand)
% Function to apply translation and rotation, and calculate forces.

% Compute new tri coords after cog rotation and translation
centerMeanFS = offsetXYZ(center,cg);
avMeanFS     = tnorm .* [area area area];

% Compute new tri coords after cog rotation and translation
center = rotateXYZ(center,[1 0 0],x(4));
center = rotateXYZ(center,[0 1 0],x(5));
center = rotateXYZ(center,[0 0 1],x(6));
center = offsetXYZ(center,x);
center = offsetXYZ(center,cg);
% Compute new normal vectors coords after cog rotation and translation
tnorm = rotateXYZ(tnorm,[1 0 0],x(4));
tnorm = rotateXYZ(tnorm,[0 1 0],x(5));
tnorm = rotateXYZ(tnorm,[0 0 1],x(6));

% Copute area vectors
av = tnorm .* [area area area];

% Calculate the free surface
wpMeanFS=pDis(centerMeanFS,       0,AH,w,dw,wDepth,deepWaterWave,t,k,phaseRand,typeNum,rho,g);
wp      =pDis(center      ,     elv,AH,w,dw,wDepth,deepWaterWave,t,k,phaseRand,typeNum,rho,g);

% Calculate forces
f_linear   =FK(centerMeanFS,       cg,avMeanFS,wpMeanFS);
f_nonLinear=FK(center      ,x(1:3)+cg,av      ,wp      );
f = f_nonLinear-f_linear;
end

function f=pDis(center,elv,AH,w,dw,wDepth,deepWaterWave,t,k,phaseRand,typeNum,rho,g)
% Function to calculate pressure distribution
f = zeros(length(center(:,3)),1);
z=zeros(length(center(:,1)),1);
if typeNum <10
elseif typeNum <20
    f = rho.*g.*AH(1).*cos(k(1).*center(:,1)-w(1)*t);
    if deepWaterWave == 0
        z=(center(:,3)-elv).*wDepth./(wDepth+elv);
        f = f.*(cosh(k(1).*(z+wDepth))./cosh(k(1)*wDepth));
    else
        z=(center(:,3)-elv);
        f = f.*exp(k(1).*z);
    end
elseif typeNum <30
    for i=1:length(AH)
        if deepWaterWave == 0 && wDepth <= 0.5*pi/k(i)
            z=(center(:,3)-elv).*wDepth./(wDepth+elv);
            f_tmp = rho.*g.*sqrt(AH(i)*dw(i)).*cos(k(i).*center(:,1)-w(i)*t-phaseRand(i));
            f = f + f_tmp.*(cosh(k(i).*(z+wDepth))./cosh(k(i).*wDepth));
        else
            z=(center(:,3)-elv);
            f_tmp = rho.*g.*sqrt(AH(i)*dw(i)).*cos(k(i).*center(:,1)-w(i)*t-phaseRand(i));
            f = f + f_tmp.*exp(k(i).*z);
        end
    end
end
f(z>0)=0;
end

function f = FK(center,instcg,av,wp)
% Function to calculate the force and moment about the cog due to Froude-Krylov pressure
f = zeros(6,1);

% Calculate the hydrostatic pressure at each triangle center
pressureVect = [wp wp wp].*-av;

% Compute force about cog
f(1:3) = sum(pressureVect);

% Compute moment about cog
tmp1 = ones(length(center(:,1)),1);
tmp2 = tmp1*instcg';
center2cgVec = center-tmp2;

f(4:6)= sum(cross(center2cgVec,pressureVect));
end

== matlab function OSWEC/Flap/Hydrodynamic Body/Wave Radiation Forces Calculation/SS CI and Constant-Damping-CoeVariant Subsystem/Convolution Integral Calculation/MATLAB Function1 ==
  data: velocity input; F_FM output; IRKB input; CTTime input
function F_FM = ConvolutionIntegral_interp(velocity, IRKB, CTTime)
%#codegen
% Function to calculate convolution integral. velocity is the only dynamic input.
% IRKB, nDOF and CTTime do not change with time.
%
% Dimensions:
% nDOF = the body's number of degrees of freedom = body.dof
% LDOF = radiating dofs from all bodies (6*Nbodies)
% nt = length of CTTime (simu.CITime / simu.dtCTTime)
%
% Paramters:
%     velocity : float [LDOF]
%         The current velocities of all bodies 
%         e.g. 6 for 1 body, 12 for 2 bodies and B2B on
% 
%     IRKB : float [nt nDOF LDOF]
%         The body's interpolated IRF, as calculated in irfInfAddedMassAndDamping
% 
%     CTTime : float [nt]
%         All CI times
%
% Returns:
%     F_FM : float [nDOF,1]

% define persistent variables to track velocity_history over time. Others are
% persistent so that the static values only need be calculated once.
interp_factor = 1;
persistent velocity_history IRKB_interp CTTime_interp;

% If this is the first time step (i.e. velocity_history is empty), 
% define the persistent variables.
if isempty(velocity_history) 
    CTTime_interp  = CTTime(1:interp_factor:end);         % [nt] interpolate CTTime if interpolation timestep ~= 1
    velocity_history = zeros(length(CTTime_interp),length(velocity)); % [nt LDOF]
    irkb_tmp    = IRKB(1:interp_factor:end, :, :);     % [nt nDOF LDOF] interpolate IRKB if interpolation timestep ~= 1
    IRKB_interp = permute(irkb_tmp,[1 3 2]); % permute to [nt LDOF nDOF]
end 

% shift velocity_history to set the first column as the current velocity
velocity_history = circshift(velocity_history, 1, 1); % shift velocity_history by 1 in the time dimension for the new time step
velocity_history(1,:) = velocity(:)';                 % [nt LDOF], fill first row with current velocity

% Multiply velocity_history and IRKB
time_series = bsxfun(@times, IRKB_interp, velocity_history); % [nt LDOF nDOF], multiply velocity_history and K_r for CI integral

% sum the effects of all radiating dofs (LDOF) for each time and motion dof (nDOF)
tmp_s = squeeze(sum(time_series,2)); % [nt nDOF]
F_FM = squeeze(trapz(CTTime_interp,tmp_s,1)); % integrate to get the wave radiation force, [nDOF, 1]

end

== matlab function OSWEC/Flap/Hydrodynamic Body/nonLinYaw force transforms/nonLinYaw force transforms ==
  data: yawNonLin input; F_Excitation output; dispGlobal input; F_RadiationDampingLocal input; F_AddedMassLocal input; F_ExcitationLocal input; F_RadiationDamping output; F_RestoringLocal input; F_AddedMass output; F_Restoring output
function [F_Excitation, F_RadiationDamping, F_AddedMass, F_Restoring] = fYawTransforms(yawNonLin, dispGlobal, F_RadiationDampingLocal, F_AddedMassLocal, F_ExcitationLocal, F_RestoringLocal)
if yawNonLin ==1
    % transform force vectors from local frame to global frame
    rotMatYaw = [cos(dispGlobal(6)), -sin(dispGlobal(6)), 0;
                 sin(dispGlobal(6)),  cos(dispGlobal(6)), 0;
                                  0,                   0, 1];

    F_RadiationDamping = [rotMatYaw*F_RadiationDampingLocal(1:3); rotMatYaw*F_RadiationDampingLocal(4:6)];
    F_AddedMass = [rotMatYaw*F_AddedMassLocal(1:3); rotMatYaw*F_AddedMassLocal(4:6)];
    F_Excitation = [rotMatYaw*F_ExcitationLocal(1:3); rotMatYaw*F_ExcitationLocal(4:6)];
    F_Restoring = [rotMatYaw*F_RestoringLocal(1:3); rotMatYaw*F_RestoringLocal(4:6)];
else
    F_RadiationDamping = F_RadiationDampingLocal;
    F_AddedMass = F_AddedMassLocal;
    F_Excitation = F_ExcitationLocal;
    F_Restoring = F_RestoringLocal;
end
end

== matlab function OSWEC/Flap/Hydrodynamic Body/Wave Diffraction and Excitation Force Calculation/Linear Wave Excitation Force Variant Subsystem/Regular Wave NonLinear Yaw/MATLAB Function1 ==
  data: A input; w input; dofGRD input; dirGRD input; fEHRE input; fEHIM input; Fext output; fEHMD input; time input; WaveDir input; Disp input; intThresh input; prevYaw input; relYawLast output; prevCoeffMD input; prevCoeffRE input; prevCoeffIM input; coeffsLastMD output; coeffsLastRE output; coeffsLastIM output
function [Fext,relYawLast,coeffsLastMD,coeffsLastRE,coeffsLastIM] = fcn(A,w,dofGRD,dirGRD,fEHRE,fEHIM, fEHMD,time,WaveDir,Disp, intThresh, prevYaw, prevCoeffMD, prevCoeffRE, prevCoeffIM)
%#codegen
% Fext is the excitation force output, relYawLast is the angle of relative
% yaw at which that last interpolation was performed. If the current
% relative yaw angle - last interpolated > threshold, the interpolation is
% performed again. To interpolate every time step, let threshold=0. 

%initialize outputs
Fext = zeros(1,6);
relYawLast=0;
coeffsLastMD=zeros(length(w),6); % should be (1,6) for regular waves
coeffsLastRE=zeros(length(w),6);
coeffsLastIM=zeros(length(w),6);

for ii=1:length(WaveDir) % should be length=1 for regular waves
    relYaw=WaveDir(ii)-(Disp(6).*180/pi); % relative yaw angle, convert to deg
   
     % compare relYaw to available WaveDir data
        if relYaw>max(dirGRD(1,:)) % handle interpolation out of BEM range by wrapping other bound
            [~,idx]=min(dirGRD,[],2); % 
            dirGRD(:,idx)=dirGRD(:,idx)+360;
            [dirGRD,I]=sort(dirGRD,2); % grid must be in ascending order
            
        elseif relYaw<min(dirGRD(1,:))
            [~,idx]=max(dirGRD,[],2); % 
            dirGRD(:,idx)=dirGRD(:,idx)-360;
            [dirGRD,I]=sort(dirGRD,2); % grid must be in ascending order
        else
            I=1:length(dirGRD(1,:));
        end
        
    if abs(relYaw-prevYaw)>intThresh && min(abs(relYaw-dirGRD(1,:)))>intThresh% interpolate for nonlinear yaw 
       
        % performs 1D interpolation in wave direction
        fExtMDint=interpn(dofGRD,dirGRD,fEHMD(:,I(1,:)),dofGRD,relYaw*ones(size(dirGRD)));
        fExtREint=interpn(dofGRD,dirGRD,fEHRE(:,I(1,:)),dofGRD,relYaw*ones(size(dirGRD)));
        fExtIMint=interpn(dofGRD,dirGRD,fEHIM(:,I(1,:)),dofGRD,relYaw*ones(size(dirGRD)));
        
        fExtMDint=fExtMDint(:,1).';
        fExtREint=fExtREint(:,1).';
        fExtIMint=fExtIMint(:,1).';
                
        relYawLast=relYaw;
        coeffsLastMD=fExtMDint;
        coeffsLastRE=fExtREint;
        coeffsLastIM=fExtIMint;
  
   elseif min(abs(relYaw-dirGRD(1,:)))>intThresh % significant yaw is present, but close to previous value
        fExtMDint=prevCoeffMD;
        fExtREint=prevCoeffRE;
        fExtIMint=prevCoeffIM;
        
        relYawLast=prevYaw;
        coeffsLastMD=prevCoeffMD;
        coeffsLastRE=prevCoeffRE;
        coeffsLastIM=prevCoeffIM;
              
    else    % significant yaw may be is present, but nearby BEM calculated data
        [~,idx]=min(abs(relYaw-dirGRD(1,:)));
        fExtMDint=fEHMD(:,I(1,idx)).'; % maintains dimensional consistency
        fExtREint=fEHRE(:,I(1,idx)).';
        fExtIMint=fEHIM(:,I(1,idx)).';
     
        relYawLast=dirGRD(1,idx); % indices of dirGRD have already been resorted
        coeffsLastMD=fExtMDint;
        coeffsLastRE=fExtREint;
        coeffsLastIM=fExtIMint;
    end

    % regular wave excitation equation (with mean drift)
    Fext = fExtMDint*A^2 + A*fExtREint*cos(w*time)- A*fExtIMint*sin(w*time);
    

end

== matlab function OSWEC/Flap/Hydrodynamic Body/Kinematic Transforms/No B2B/nonLinYaw Kinematic transforms ==
  data: yawNonLin input; dispLoc output; dispGlobal input; velGlobal input; accGlobal input; velLoc output; accLoc output
function [dispLoc, velLoc, accLoc] = kinYawTransform(yawNonLin, dispGlobal, velGlobal, accGlobal)
if yawNonLin == 1
    % rotate kinematics to 'zero' the yaw displacement (in order to
    % calculate F_RadiationDamping, F_AddedMass and F_Restoring in the
    % local frame).
    rotMatYaw = [cos(dispGlobal(6)), -sin(dispGlobal(6)), 0;
                 sin(dispGlobal(6)),  cos(dispGlobal(6)), 0;
                                  0,                   0, 1];

    rotMatYawTranspose = rotMatYaw.';
    rotMatGlobal = eulXYZ2RotMat(dispGlobal(4), dispGlobal(5), dispGlobal(6));
    rotMatLoc = rotMatYawTranspose*rotMatGlobal;

    [phiLoc, thetaLoc, psiLoc] = rotMatXYZ2Eul(rotMatLoc);
    dispLoc = [rotMatYawTranspose*dispGlobal(1:3); phiLoc; thetaLoc; psiLoc];
    velLoc = [rotMatYawTranspose*velGlobal(1:3); rotMatYawTranspose*velGlobal(4:6)];
    accLoc = [rotMatYawTranspose*accGlobal(1:3); rotMatYawTranspose*accGlobal(4:6)];
else
    dispLoc = dispGlobal;
    velLoc = velGlobal;
    accLoc = accGlobal;
end
end

== matlab function OSWEC/Flap/Hydrodynamic Body/Kinematic Transforms/With B2B/MATLAB Function ==
  data: yawNonLin input; dispLoc output; dispGlobal input; velGlobal input; accGlobal input; velLoc output; accLoc output; numBody parameter
function [dispLoc, velLoc, accLoc] = kinYawTransform(yawNonLin, dispGlobal, velGlobal, accGlobal, numBody)

% pre-allocate outputs
    dispLoc=zeros(6,1);
    velLoc=zeros(numBody*6,1);
    accLoc=zeros(numBody*6,1);
    
if yawNonLin == 1
    % rotate kinematics to 'zero' the yaw displacement (in order to
    % calculate F_RadiationDamping, F_AddedMass and F_Restoring in the
    % local frame).
            
    rotMatYaw = [cos(dispGlobal(6)), -sin(dispGlobal(6)), 0;
                 sin(dispGlobal(6)),  cos(dispGlobal(6)), 0;
                                  0,                   0, 1];

    rotMatYawTranspose = rotMatYaw.';
    rotMatGlobal = eulXYZ2RotMat(dispGlobal(4), dispGlobal(5), dispGlobal(6));
    rotMatLoc = rotMatYawTranspose*rotMatGlobal;

    [phiLoc, thetaLoc, psiLoc] = rotMatXYZ2Eul(rotMatLoc);
    dispLoc = [rotMatYawTranspose*dispGlobal(1:3); phiLoc; thetaLoc; psiLoc];
   for k=1:length(velGlobal)/6 % loop through each 6-dof body
        velLoc(6*(k-1)+1:6*(k-1)+6) = [rotMatYawTranspose*velGlobal((6*(k-1)+1):(6*(k-1)+3));...
            rotMatYawTranspose*velGlobal((6*(k-1)+4):(6*(k-1)+6))];
        accLoc(6*(k-1)+1:6*(k-1)+6) = [rotMatYawTranspose*accGlobal((6*(k-1)+1):(6*(k-1)+3));...
            rotMatYawTranspose*accGlobal((6*(k-1)+4):(6*(k-1)+6))];
    end
else
    dispLoc = dispGlobal;
    velLoc = velGlobal;
    accLoc = accGlobal;
end
end
